simulink model "MainPendulum"  (R2021b)
settings: Solver=VariableStepAuto  StartTime=0.0  StopTime=20.0  RelTol=1e-3
values from neighbouring files (symbols this model uses):
  h = 0.01    [build_sysid_parameters.m]
undefined symbols (not defined in the file or in its folder): adingain, adinoffs, daoutgain, daoutoffs, Discrete, Kx, Time
libraries: ctrlSharedLib x1
settings Model: Creator=djangovanderplas  LastModifiedBy=tsderksen
settings DebuggingCC: UnconnectedInputMsg=none  UnconnectedOutputMsg=none  UnconnectedLineMsg=none
settings ModelReferenceCC: EnableRefExpFcnMdlSchedulingChecks=off
settings RTWCC: GPUComputeCapability=5.0  DLArmComputeVersion=20.02.1

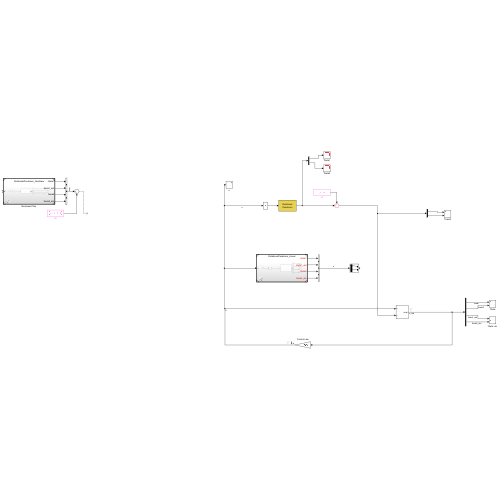
[thumbnail: Simulink's stored preview of the top-level diagram]
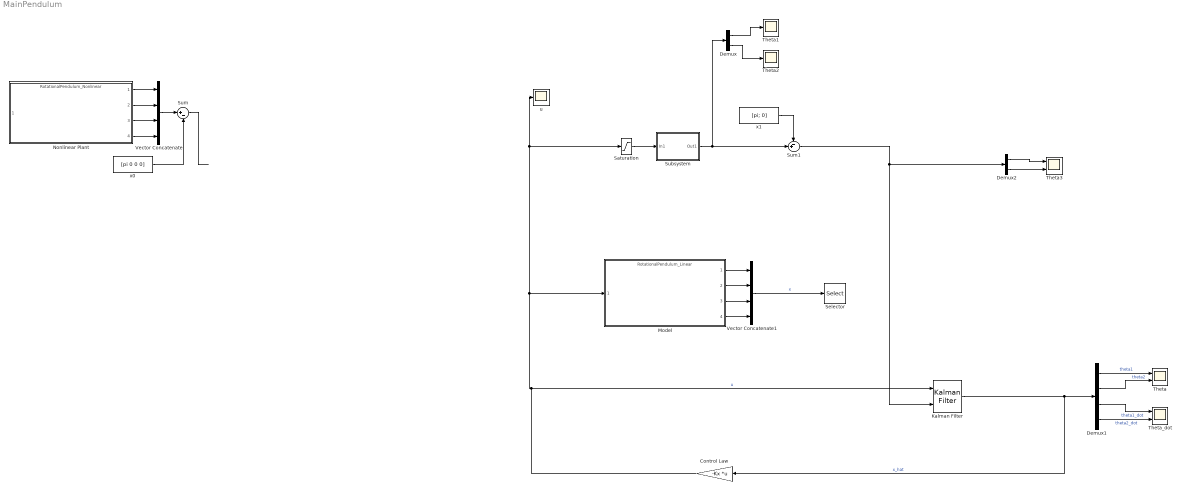
== system MainPendulum ==
  Control Law : Gain  Gain=-Kx  Multiplication=Matrix(K*u)
  Demux : Demux  Outputs=2
  Demux1 : Demux
  Demux2 : Demux  Outputs=2
  Kalman Filter : ctrlSharedLib/Kalman Filter  TimeDomain=Discrete-Time  UseCurrentEstimator=on  ModelSource=LTI State-Space Variable  ModelSourceVariable=sys_kf_d  A=0.95  B=1  C=1  D=0  NumberOfStates=1  NumberOfInputs=1  NumberOfOutputs=1  InitialEstimateSource=Dialog  X0=[0 0 0 0]  P0=10  UseK=off  UseGH=off  NumberOfProcessNoiseInputs=1  G=1  TimeInvariantG=on  H=0  TimeInvariantH=on  Q=0.8*eye(4)  TimeInvariantQ=on  R=[7.335173479896564e-06, 0; 0, 1.134946947651487e-05]  TimeInvariantR=on  N=zeros(4, 2)  TimeInvariantN=on  AddInputPort=on  AddEnablePort=off  OutputEstimatedY=off  OutputP=off  Ts=-1
  Model : ModelReference  ModelNameDialog=RotationalPendulum_Linear.slx  SimulationMode=Normal  ModelReferenceVersion=1.2
  Nonlinear Plant : ModelReference  ModelNameDialog=RotationalPendulum_Nonlinear  SimulationMode=Normal  ModelReferenceVersion=1.0
  Saturation : Saturate  UpperLimit=1  LowerLimit=-1
  Selector : Selector  InputPortWidth=4  IndexOptions=Index vector (dialog)  Indices=[1 3]  OutputSizes=1
  Subsystem : Subsystem
      mask Display: disp('Rotational\nPendulum')
  Sum : Sum  Inputs=|+-
  Sum1 : Sum  Inputs=-+|
  Theta : Scope  NumInputPorts=2
  Theta1 : Scope
  Theta2 : Scope
  Theta3 : Scope  NumInputPorts=2
  Theta_dot : Scope  NumInputPorts=2
  Vector Concatenate : Concatenate  NumInputs=4
  Vector Concatenate1 : Concatenate  NumInputs=4
  u : Scope
  x0 : Constant  Value=[pi 0 0 0]
  x1 : Constant  Value=[pi; 0]  SampleTime=h
  wires:
  Nonlinear Plant/1 -> Vector Concatenate/1
  Nonlinear Plant/2 -> Vector Concatenate/2
  Nonlinear Plant/3 -> Vector Concatenate/3
  Nonlinear Plant/4 -> Vector Concatenate/4
  Model/1 -> Vector Concatenate1/1
  Model/2 -> Vector Concatenate1/2
  Model/3 -> Vector Concatenate1/3
  Model/4 -> Vector Concatenate1/4
  Vector Concatenate/1 -> Sum/1
  Sum/1 -> ?
  Vector Concatenate1/1 -> Selector/1  "x"
  x0/1 -> Sum/2
  Control Law/1 -> u/1, Saturation/1, Model/1, Kalman Filter/1  "u"
  Demux/1 -> Theta1/1
  Saturation/1 -> Subsystem/1(In1)
  Demux/2 -> Theta2/1
  Subsystem/1(Out1) -> Demux/1, Sum1/2
  x1/1 -> Sum1/1
  Sum1/1 -> Demux2/1, Kalman Filter/2
  Kalman Filter/1 -> Demux1/1, Control Law/1  "x_hat"
  Demux1/1 -> Theta/1  "theta1"
  Demux1/3 -> Theta_dot/1  "theta1_dot"
  Demux1/2 -> Theta/2  "theta2"
  Demux1/4 -> Theta_dot/2  "theta2_dot"
  Demux2/1 -> Theta3/1
  Demux2/2 -> Theta3/2

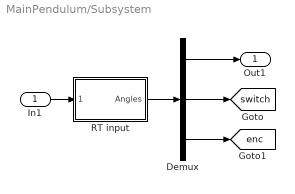
== system MainPendulum/Subsystem ==
  In1 : Inport
  Demux : Demux  Outputs=[2 4 1]
  RT input : Subsystem  mask{Ts=h, channels=[6 7]}
      mask prompts: Ts "Sample time [s]:"; channels "Channels to read (e.g., [6 7])"
      mask init:
      | hwinit;
      | 
      | % initialize FPGA
      | fugihandle = fugiboard('Open', 'Pendulum1');
      | fugihandle.WatchdogTimeout = 0.5;
      | fugiboard('SetParams', fugihandle);
      | fugiboard('Write', fugihandle, 0, 0, 0, 0);  % dummy write to sync interface board
      | fugiboard('Write', fugihandle, 5, 1, 0, 0);  % reset position, activate relay
      | data = fugiboard('Read', fugihandle);        % get version info from FPGA
      | % model = bitshift(data(1), -5); 
      | % version = bitand(data(1), 31);
      | % disp(sprintf('FPGA setup %d, version %d', model, version)); % for the B&P it should say 1 1, or else there is a problem
      | fugiboard('Write', fugihandle, 0, 1, 0, 0);  % end reset
      | pause(0.1);                         % give relay some time to respond
      mask Display: disp('Rotational\nPendulum')
  Out1 : Outport
  tag scope: enc=global, switch=global
  wires:
  RT input/1(Angles) -> Demux/1
  Demux/1 -> Out1/1
  Demux/2 -> [switch]
  Demux/3 -> [enc]
  In1/1 -> RT input/1(Motors)

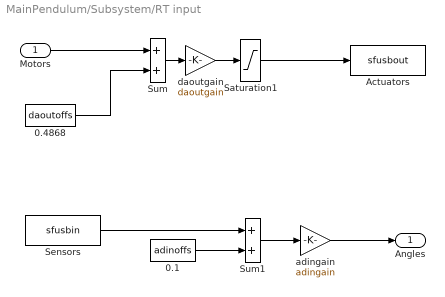
== system MainPendulum/Subsystem/RT input ==
  Motors : Inport
  0.1 : Constant  Value=adinoffs
  0.4868 : Constant  Value=daoutoffs
  Actuators : S-Function  FunctionName=sfusbout  Parameters=Ts, fugihandle  SFunctionDeploymentMode=off  EnableBusSupport=off
  Saturation1 : Saturate  UpperLimit=10  LowerLimit=-10
  Sensors : S-Function  FunctionName=sfusbin  Parameters=Ts, fugihandle, channels  SFunctionDeploymentMode=off  EnableBusSupport=off
  Sum : Sum  InputSameDT=on  SaturateOnIntegerOverflow=on  OutDataTypeStr=Inherit: Same as first input
  Sum1 : Sum  InputSameDT=on  SaturateOnIntegerOverflow=on  OutDataTypeStr=Inherit: Same as first input
  adingain : Gain  Gain=adingain  SaturateOnIntegerOverflow=on  OutDataTypeStr=Inherit: Same as input  ParamDataTypeStr=Inherit: Same as input
  daoutgain : Gain  Gain=daoutgain  SaturateOnIntegerOverflow=on  OutDataTypeStr=Inherit: Same as input  ParamDataTypeStr=Inherit: Same as input
  Angles : Outport
  wires:
  Sum/1 -> daoutgain/1
  0.4868/1 -> Sum/2
  Motors/1 -> Sum/1
  Sum1/1 -> adingain/1
  0.1/1 -> Sum1/2
  adingain/1 -> Angles/1
  Saturation1/1 -> Actuators/1
  daoutgain/1 -> Saturation1/1
  Sensors/1 -> Sum1/1
